simulink model "simulation_poursuite"  (Simulink 7.7)
settings: Solver=ode45  StartTime=0.0  StopTime=2  RelTol=1e-6
values from neighbouring files (symbols this model uses):
  bruit_bf = 0    [PetitGain24V.m]
  consigne_bf = 1    [PetitGain24V.m]
  pertu_entree_bf = 0    [PetitGain24V.m]
  pertu_sortie_bf = 1    [PetitGain24V.m]
undefined symbols (not defined in the file or in its folder): Rd_tf
libraries: cstblocks x6
settings Model: Creator=adminportog  LastModifiedBy=Nicolas
settings OptimizationCC: InitFltsAndDblsToZero=on
settings DebuggingCC: StrictBusMsg=Warning

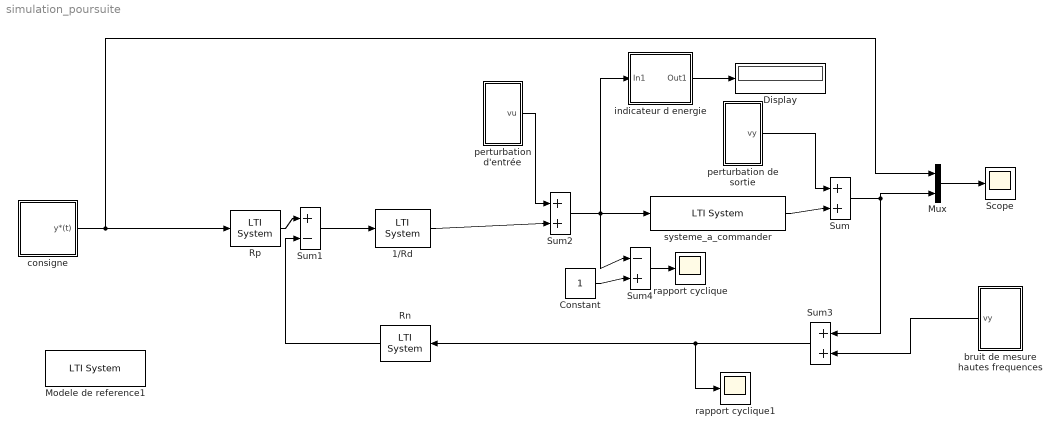
== system simulation_poursuite ==
  1/Rd : cstblocks/LTI System  SystemSampleTime=-1  sys=1/Rd_tf  IC=[]
  Constant : Constant
  Display : Display
  Modele de reference1 : cstblocks/LTI System  SystemSampleTime=-1  sys=modele_reference  IC=[]
  Mux : Mux  Inputs=2
  Rn : cstblocks/LTI System  SystemSampleTime=-1  sys=Rn_tf  IC=[]
  Rp : cstblocks/LTI System  SystemSampleTime=-1  sys=Rp_tf  IC=[]
  Scope : Scope
      settings: TimeRange=0.3857142857142856  YMin=0  YMax=27.5  MaxDataPoints=50000
  Sum : Sum  Inputs=|++
  Sum1 : Sum  Inputs=|+-
  Sum2 : Sum  Inputs=|++
  Sum3 : Sum
  Sum4 : Sum  Inputs=|-+
  bruit de mesure hautes frequences : Subsystem
  consigne : Subsystem
  indicateur d energie : Subsystem
  perturbation d'entrée : Subsystem
  perturbation de sortie : Subsystem
  rapport cyclique : Scope
      settings: YMin=0.52045  YMax=0.52115  MaxDataPoints=50000
  rapport cyclique1 : Scope
      settings: YMin=-0.11  YMax=0.11  SaveName=ScopeData2  MaxDataPoints=50000
  systeme_a_commander : cstblocks/LTI System  SystemSampleTime=-1  sys=G_nominal_commande  IC=[]
  wires:
  systeme_a_commander/1 -> Sum/2
  Sum/1 -> Mux/2, Sum3/1
  Sum1/1 -> 1/Rd/1
  Rn/1 -> Sum1/2
  Rp/1 -> Sum1/1
  Mux/1 -> Scope/1
  indicateur d energie/1(Out1) -> Display/1
  perturbation de sortie/1(vy) -> Sum/1
  Sum2/1 -> systeme_a_commander/1, indicateur d energie/1(In1), Sum4/1
  perturbation d'entrée/1(vu) -> Sum2/1
  Sum3/1 -> rapport cyclique1/1, Rn/1
  bruit de mesure hautes frequences/1(vy) -> Sum3/2
  Sum4/1 -> rapport cyclique/1
  Constant/1 -> Sum4/2
  consigne/1(y*(t)) -> Rp/1, Mux/1
  1/Rd/1 -> Sum2/2

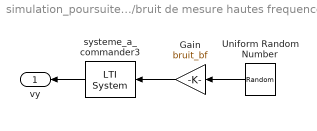
== system simulation_poursuite/bruit de mesure hautes frequences ==
  Gain : Gain  Gain=bruit_bf
  Uniform Random Number : UniformRandomNumber  Minimum=-0.1  Maximum=0.1  SampleTime=0
  systeme_a_commander3 : cstblocks/LTI System  SystemSampleTime=-1  sys=tf([1 8*1e4],[1 1e5])  IC=[]
  vy : Outport
  wires:
  Gain/1 -> systeme_a_commander3/1
  systeme_a_commander3/1 -> vy/1
  Uniform Random Number/1 -> Gain/1

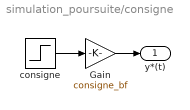
== system simulation_poursuite/consigne ==
  Gain : Gain  Gain=consigne_bf
  consigne : Step  After=24  SampleTime=0
  y*(t) : Outport
  wires:
  consigne/1 -> Gain/1
  Gain/1 -> y*(t)/1

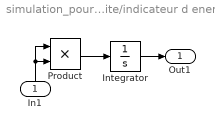
== system simulation_poursuite/indicateur d energie ==
  In1 : Inport
  Integrator : Integrator
  Product : Product  RndMeth=Zero
  Out1 : Outport
  wires:
  Product/1 -> Integrator/1
  In1/1 -> Product/2, Product/1
  Integrator/1 -> Out1/1

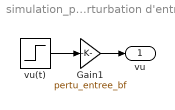
== system simulation_poursuite/perturbation d'entrée ==
  Gain1 : Gain  Gain=pertu_entree_bf
  vu(t) : Step  Time=1.8  After=0.3  SampleTime=0
  vu : Outport
  wires:
  Gain1/1 -> vu/1
  vu(t)/1 -> Gain1/1

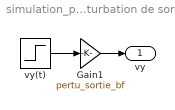
== system simulation_poursuite/perturbation de sortie ==
  Gain1 : Gain  Gain=pertu_sortie_bf
  vy(t) : Step  Time=1.5  SampleTime=0
  vy : Outport
  wires:
  vy(t)/1 -> Gain1/1
  Gain1/1 -> vy/1
